simulink model "Utensile"  (R2019a)
settings: Solver=VariableStepAuto  StartTime=0.0  StopTime=10.0  RelTol=1e-3
settings Model: Creator=anton  LastModifiedBy=anton

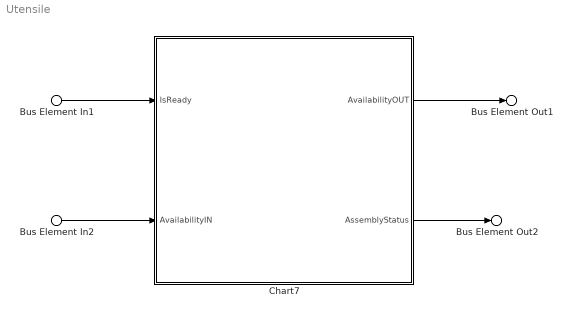
== system Utensile ==
  Bus Element In1 : Inport  PortName=IsReady
  Bus Element In2 : Inport  Port=2  PortName=AvailabilityIN
  Chart7 : Stateflow chart  BlockKeywords=__PRM__SERIALIZED__DATA__:Stateflow Chart,Stateflow Diagram  TreatAsAtomicUnit=on
  Bus Element Out1 : Outport  PortName=AvailabilityOUT
  Bus Element Out2 : Outport  Port=2  PortName=AssemblyStatus
  wires:
  Bus Element In1/1 -> Chart7/1(IsReady)
  Chart7/1(AvailabilityOUT) -> Bus Element Out1/1
  Chart7/2(AssemblyStatus) -> Bus Element Out2/1
  Bus Element In2/1 -> Chart7/2(AvailabilityIN)

== stateflow chart Utensile/Chart7 ==
  state CheckDisponibility
    if IsReady == 1 && AvailabilityIN == 1
    AvailabilityOUT = AvailabilityIN;
    AssemblyStatus = 1;
    end
  (default) -> CheckDisponibility
  data: IsReady input; AvailabilityIN input; AvailabilityOUT output; AssemblyStatus output
